simulink model "may7bdrc"  (Simulink 8.5)
settings: Solver=ode4  StartTime=0.0  StopTime=inf  FixedStep=BKIN_STEP_TIME  RelTol=1e-3
StartFcn:
  |  warndlg('Dexterit-E models cannot run under simulation. Please compile your model and run it from within Dexterit-E.');set_param(bdroot,'SimulationCommand','stop')
undefined symbols (not defined in the file): slselsubs
libraries: Video x7, General x3, KINARM_loads x2, KINARM_EP_loads x1, KINARM_general x1, simulink x1, slrtlib x1
(part 2 of 3)

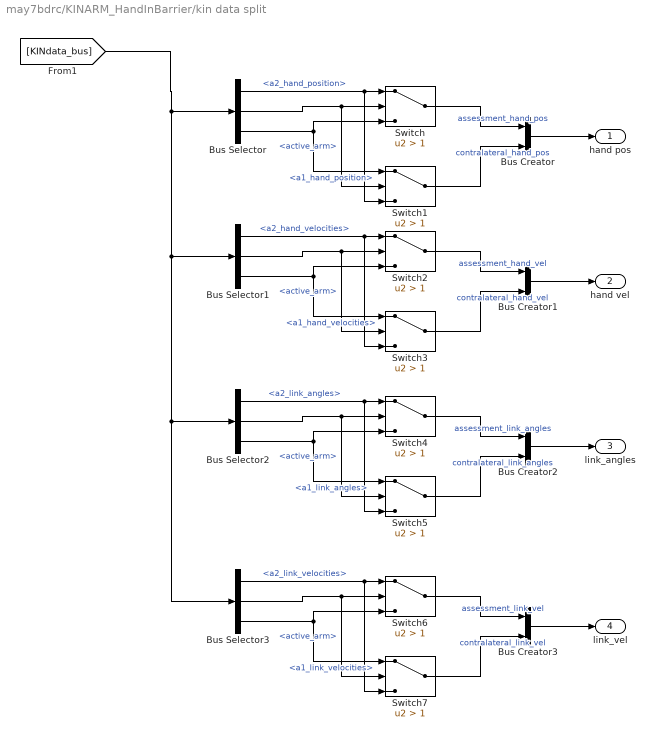
== system may7bdrc/KINARM_HandInBarrier/kin data split ==
  Bus Creator{,1..3} (4 alike) : BusCreator  Inputs=2
  Bus Selector : BusSelector  OutputSignals=Robot2.a2_hand_position,KINDataGeneral.active_arm,Robot1.a1_hand_position
  Bus Selector1 : BusSelector  OutputSignals=Robot2.a2_hand_velocities,KINDataGeneral.active_arm,Robot1.a1_hand_velocities
  Bus Selector2 : BusSelector  OutputSignals=Robot2.a2_link_angles,KINDataGeneral.active_arm,Robot1.a1_link_angles
  Bus Selector3 : BusSelector  OutputSignals=Robot2.a2_link_velocities,KINDataGeneral.active_arm,Robot1.a1_link_velocities
  Switch{,1..7} (8 alike) : Switch  Criteria=u2 > Threshold  Threshold=1
  hand pos : Outport
  hand vel : Outport  Port=2
  link_angles : Outport  Port=3
  link_vel : Outport  Port=4
  wires:
  Bus Selector/1 -> Switch1/3, Switch/1  "<a2_hand_position>"
  Switch/1 -> Bus Creator/1  "assessment_hand_pos"
  Switch1/1 -> Bus Creator/2  "contralateral_hand_pos"
  Bus Creator/1 -> hand pos/1
  Bus Selector/3 -> Switch1/1, Switch/3  "<a1_hand_position>"
  Bus Selector/2 -> Switch1/2, Switch/2  "<active_arm>"
  Bus Selector1/1 -> Switch3/3, Switch2/1  "<a2_hand_velocities>"
  Switch2/1 -> Bus Creator1/1  "assessment_hand_vel"
  Switch3/1 -> Bus Creator1/2  "contralateral_hand_vel"
  Bus Creator1/1 -> hand vel/1
  Bus Selector1/3 -> Switch3/1, Switch2/3  "<a1_hand_velocities>"
  Bus Selector1/2 -> Switch3/2, Switch2/2  "<active_arm>"
  Bus Selector2/1 -> Switch5/3, Switch4/1  "<a2_link_angles>"
  Switch4/1 -> Bus Creator2/1  "assessment_link_angles"
  Switch5/1 -> Bus Creator2/2  "contralateral_link_angles"
  Bus Creator2/1 -> link_angles/1
  Bus Selector2/3 -> Switch5/1, Switch4/3  "<a1_link_angles>"
  Bus Selector2/2 -> Switch5/2, Switch4/2  "<active_arm>"
  Bus Selector3/1 -> Switch7/3, Switch6/1  "<a2_link_velocities>"
  Switch6/1 -> Bus Creator3/1  "assessment_link_vel"
  Switch7/1 -> Bus Creator3/2  "contralateral_link_vel"
  Bus Creator3/1 -> link_vel/1
  [KINdata_bus] -> Bus Selector3/1, Bus Selector2/1, Bus Selector1/1, Bus Selector/1
  Bus Selector3/3 -> Switch7/1, Switch6/3  "<a1_link_velocities>"
  Bus Selector3/2 -> Switch7/2, Switch6/2  "<active_arm>"

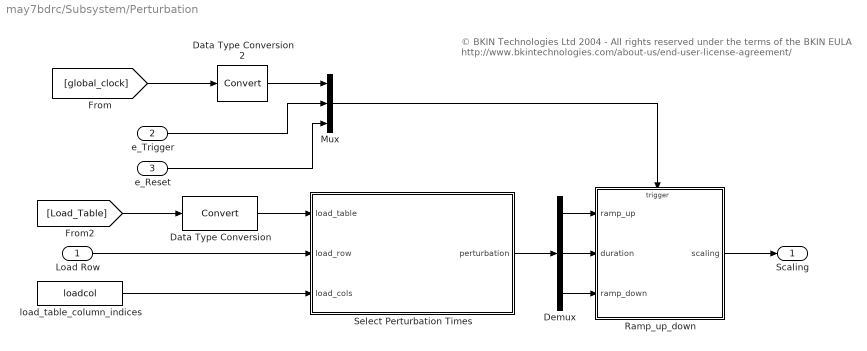
== system may7bdrc/Subsystem/Perturbation ==
  note: © BKIN Technologies Ltd 2004  - All rights reserved under the terms of the BKIN EULA
      | http://www.bkintechnologies.com/about-us/end-user-license-agreement/
  Load Row : Inport
  e_Trigger : Inport  Port=2
  e_Reset : Inport  Port=3
  Data Type Conversion : DataTypeConversion
  Data Type Conversion2 : DataTypeConversion
  Demux : Demux  Outputs=3
  Mux : Mux  Inputs=3
  Ramp_up_down : Stateflow chart  TreatAsAtomicUnit=on
      settings: PermitHierarchicalResolution=ParametersOnly
  Select Perturbation Times : MATLAB Function  TreatAsAtomicUnit=on
      settings: PermitHierarchicalResolution=ParametersOnly
  load_table_column_indices : Constant  Value=loadcol
  Scaling : Outport
  wires:
  Data Type Conversion2/1 -> Mux/1
  Mux/1 -> Ramp_up_down/Trigger
  Demux/3 -> Ramp_up_down/3(ramp_down)
  Demux/2 -> Ramp_up_down/2(duration)
  Demux/1 -> Ramp_up_down/1(ramp_up)
  [global_clock] -> Data Type Conversion2/1
  Ramp_up_down/1(scaling) -> Scaling/1
  e_Trigger/1 -> Mux/2
  e_Reset/1 -> Mux/3
  [Load_Table] -> Data Type Conversion/1
  Load Row/1 -> Select Perturbation Times/2(load_row)
  load_table_column_indices/1 -> Select Perturbation Times/3(load_cols)
  Select Perturbation Times/1(perturbation) -> Demux/1
  Data Type Conversion/1 -> Select Perturbation Times/1(load_table)

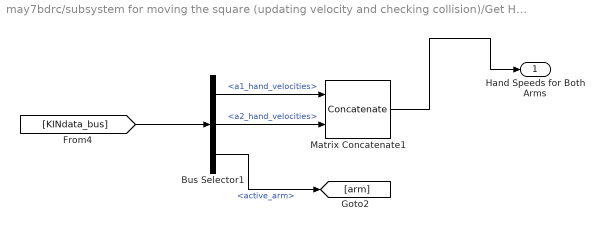
== system may7bdrc/subsystem for moving the square (updating velocity and checking collision)/Get Hand Speed ==
  Bus Selector1 : BusSelector  OutputSignals=Robot1.a1_hand_velocities,Robot2.a2_hand_velocities,KINDataGeneral.active_arm
  Matrix Concatenate1 : Concatenate  Mode=Multidimensional array
  Hand Speeds for Both Arms : Outport
  wires:
  [KINdata_bus] -> Bus Selector1/1
  Bus Selector1/1 -> Matrix Concatenate1/1  "<a1_hand_velocities>"
  Matrix Concatenate1/1 -> Hand Speeds for Both Arms/1
  Bus Selector1/2 -> Matrix Concatenate1/2  "<a2_hand_velocities>"
  Bus Selector1/3 -> [arm]  "<active_arm>"

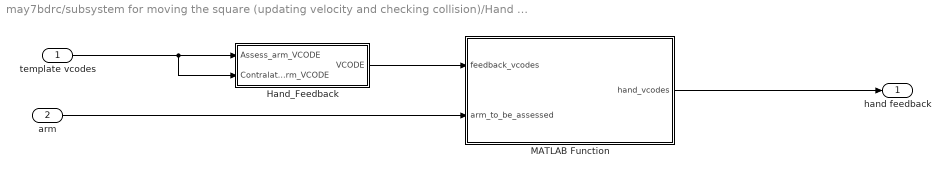
== system may7bdrc/subsystem for moving the square (updating velocity and checking collision)/Hand Feedback ==
  template vcodes : Inport
  arm : Inport  Port=2
  Hand_Feedback : Subsystem  AncestorBlock=KINARM_general/Hand_Feedback  mask(Hand_Feedback){feedback_cntl_src=style and status}
      mask prompts: feedback_cntl_src "Task Program control of style and status"
      mask help:
      | This block controls various options for hand feedback (i.e. fingertip position)  to be shown to the subject.
      |
      | Task Program control of style and status refers to whether the Program Task will explicity control the style and/or status of the hand feedback.
      mask init:
      | block_path = gcb;  % store block path, as gcb may change with block operations
      | 
      | %%% Handle background colours if link status changes.  
      | checkBackgroundColour(block_path, 'KINARM_general');
      | 
      | 
      | feedback_cntl_source=get_param(gcb,'feedback_cntl_src');
      | 
      | if feedback_cntl_source(1:4)=='none'
      |     block1type='Constant';
      |     block2type='Constant';
      |     block3type='Constant';
      | elseif feedback_cntl_source(1:4)=='stat'
      |     block1type='Constant';
      |     block2type='Constant';
      |     block3type='Inport';
      | else 
      |     block1type='Inport';
      |     block2type='Inport';
      |     block3type='Constant';
      | end
      | 
      | hasOldName1 = ~isempty(find_system(gcb, 'FollowLinks', 'on', 'LookUnderMasks', 'all', 'name', 'Dom_VCODE'));
      | hasOldName2 = ~isempty(find_system(gcb, 'FollowLinks', 'on', 'LookUnderMasks', 'all', 'name', 'non-Dom_VCODE'));
      | 
      | block1name='Assess_arm_VCODE';
      | block2name='Contralateral_arm_VCODE';
      | block1path=[gcb '/' block1name];
      | block2path=[gcb '/' block2name];
      | 
      | if hasOldName1
      | 	set_param([gcb '/Dom_VCODE'],'name', block1name);
      | end
      | 
      | if hasOldName2
      | 	set_param([gcb '/non-Dom_VCODE'],'name', block2name);
      | end
      | 
      | if ~strcmp(get_param(block1path,'blocktype'),block1type)
      | 	pos=get_param(block1path,'position');
      | 	delete_line(gcb, [block1name '/1'], 'Reshape/1');
      | 	delete_block(block1path);
      | 	add_block(['built-in/' block1type], block1path,'Name',block1name);
      | 	set_param(block1path,'position',pos);
      | 	add_line(gcb, [block1name '/1'], 'Reshape/1');
      | end
      | 
      | if ~strcmp(get_param(block2path,'blocktype'),block2type)
      | 	pos=get_param(block2path,'position');
      | 	delete_line(gcb, [block2name '/1'], 'Reshape1/1');
      | 	delete_block(block2path);
      | 	add_block(['built-in/' block2type],block2path,'Name',block2name);
      | 	set_param(block2path,'position',pos);
      | 	add_line(gcb, [block2name '/1'], 'Reshape1/1');
      | end
      | 
      | block3name='feedback_status';
      | block3path=[gcb '/' block3name];
      | if ~strcmp(get_param(block3path,'blocktype'),block3type)
      | 	pos=get_param(block3path,'position');
      | 	delete_line(gcb, [block3name '/1'], 'FeedFwdArm/3');
      | 	delete_block(block3path);
      | 	add_block(['built-in/' block3type],block3path,'Name',block3name);
      | 	set_param(block3path,'position',pos);
      | 	add_line(gcb, [block3name '/1'], 'FeedFwdArm/3');
      | end
      | 
      | if feedback_cntl_source(1:4)=='none'
      | 	set_param(block1path,'Value','[1:70]');
      | 	set_param(block2path,'Value','[71:140]');
      | elseif feedback_cntl_source(1:4)=='stat'
      | 	set_param(block1path,'Value','[1:70]');
      | 	set_param(block2path,'Value','[71:140]');
      | end
      mask Help:
      | Creates VCODE for drawing hand position (fingertip).
      | <P>
      | <H2>Library </H2>
      | KINARM general
      | 
      | <H2>Description </H2>
      | This block controls various options for drawing hand feedback.  (Note: although it is called hand feedback, it is actually the fingertip position that is shown).  Three options are available (as chosen in the Parameters and Dialog box):
      | <P>
      | (i) GUI control of feedback style and status
      | <Blockquote>
      | No inputs are required for this option.  The Task Program has no control over the style or status of the hand feedback.
      | </Blockquote>
      | (ii) Task Program control of feedback status and GUI control of style
      | <Blockquote>
      | If Task Program control of feedback status is chosen, then one input appears for this block:<P>
      | <B> feedback_status: </B> this scalar input dynamically controls the status of the hand feedback as per the following:
      | <P>
      | 0 = (no hand feedback)<BR>
      | 1 = ("arm to be assessed" hand feedback only)<BR>
      | 2 = (contralateral arm hand feedback only)<BR>
      | 3 = (hand feedback on for both hands)<BR>
      | </Blockquote>
      | (iii) Task Program control of both feedback style and status.
      | <Blockquote>
      | 
      | If Task Program control of feedback status and style is chosen, then two inputs appear for this block:<P>
      | <B> Assess_arm_VCODE: </B>  this vector input dynamically controls the status and style of the hand feedback for the "arm to be assessed" the operator selected in Dexterit-E.
      | <P>
      | <B> Contralateral_arm_VCODE:</B>  this vector input dynamically controls the status and style of the hand feedback for the contralateral hand.
      | <P>
      | For both the Assess_arm_VCODE and the Contralateral_arm_VCODE, the input vectors must be in the appropriate VCODE format (for more information on the details of a VCODE, please right click on the Show_Target block in the video library, "Look Under Mask" and open the Embedded Matlab function).  Note that the position information in the Dom_VCODE and non-Dom_VCODE are overwritten in this block, but all other aspects of the VCODE are passed through to the output.
      | </Blockquote>
      | Note that if Task Program control is chosen for either hand feedback status or style, the GUI will still override these settings if the Task Protocol specifies that it should do so.
      | <P>
      | There is one output from this block:
      | <P>
      | <B> VCODE: </B> this output is 2-row matrix containing 2 VCODEs.  The first VCODE is for the dominant hand feedback and the second VCODE is for the non-dominant hand feedback.  This output must go to the Process_Video_CMD block of the video library for the hand feedback to actually be shown (if any other visual targets are to be displayed, then this VCODE output must be concatenated with the other VCODES prior to connection to the Process_Video_CMD block - see Help for the Process_Video_CMD block for more information).
      | <H2>Parameters and Dialog Box</H2>
      | <B>Task Program control of style and status</B> refers to whether the Program Task will explicity control the style and/or status of the hand feedback.  The three options are: none, status only, or status and style.
      | <P>
      |  - Choosing none means that style and status are always controlled by the GUI.
      | <P>
      |  - Choosing status only means that the GUI always controls the hand feedback style, but also will create an input to this block allowing the end user to control the status dynamically.  Allowable input values are: 0 (no hand feedback), 1 (dominant hand feedback only), 2 (non-dominant hand feedback only) or 3 (hand feedback on for both hands)
      |  <P>
      | - Choosing status and style means that both the hand feedback status and style can be controlled dynamically by the Task Program.  If this option is selected, then two inputs will be created for this block: dominant VCODE and non-dominant VCODE.  These two inputs require a proper VCODE (e.g. from a Show_Target block) for each.  Because status and style are both part of a VCODE, there is no separate input for hand feedback status.  Note: any position information of these input VCODEs is overwritten by this block by the appropriate fingertip locations.
      | <P>
      | 
      | <H2>Related Blocks </H2>
      | DataLogging<BR>
      | Show_Target<BR>
      | Process_Video_CMD
      mask TypeOptions feedback_cntl_src: none | status only | style and status
  MATLAB Function : MATLAB Function  TreatAsAtomicUnit=on
      settings: PermitHierarchicalResolution=ParametersOnly
  hand feedback : Outport
  wires:
  template vcodes/1 -> Hand_Feedback/2(Contralateral_arm_VCODE), Hand_Feedback/1(Assess_arm_VCODE)
  Hand_Feedback/1(VCODE) -> MATLAB Function/1(feedback_vcodes)
  arm/1 -> MATLAB Function/2(arm_to_be_assessed)
  MATLAB Function/1(hand_vcodes) -> hand feedback/1

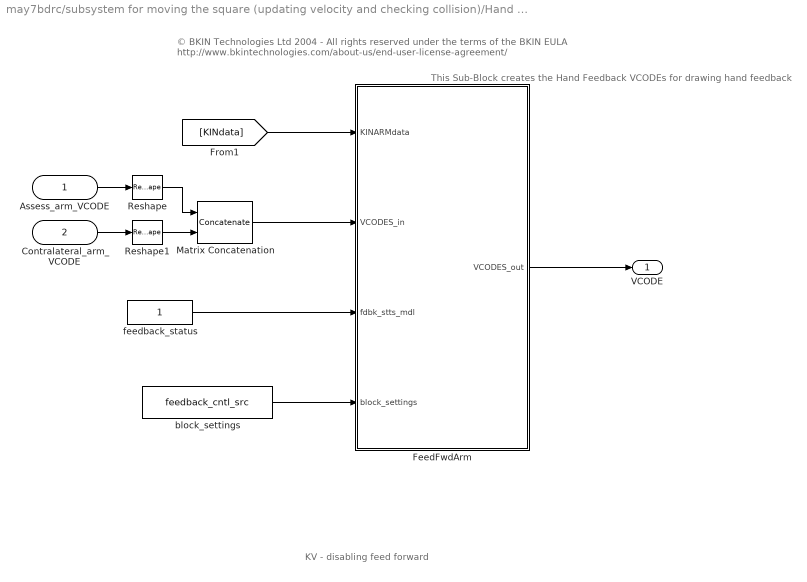
== system may7bdrc/subsystem for moving the square (updating velocity and checking collision)/Hand Feedback/Hand_Feedback ==
  note: KV - disabling feed forward
  note: This Sub-Block creates the Hand Feedback VCODEs for drawing hand feedback
  note: © BKIN Technologies Ltd 2004  - All rights reserved under the terms of the BKIN EULA
      | http://www.bkintechnologies.com/about-us/end-user-license-agreement/
  Assess_arm_VCODE : Inport
  Contralateral_arm_VCODE : Inport  Port=2
  FeedFwdArm : MATLAB Function  TreatAsAtomicUnit=on
      settings: PermitHierarchicalResolution=ParametersOnly  RTWSystemCode=Nonreusable function  RTWFileNameOpts=Use function name
  Matrix Concatenation : Concatenate  Mode=Multidimensional array
  Reshape : Reshape  OutputDimensionality=Row vector (2-D)
  Reshape1 : Reshape  OutputDimensionality=Row vector (2-D)
  block_settings : Constant  Value=feedback_cntl_src
  feedback_status : Constant
  VCODE : Outport
  wires:
  feedback_status/1 -> FeedFwdArm/3(fdbk_stts_mdl)
  FeedFwdArm/1(VCODES_out) -> VCODE/1
  block_settings/1 -> FeedFwdArm/4(block_settings)
  Matrix Concatenation/1 -> FeedFwdArm/2(VCODES_in)
  [KINdata] -> FeedFwdArm/1(KINARMdata)
  Reshape1/1 -> Matrix Concatenation/2
  Reshape/1 -> Matrix Concatenation/1
  Assess_arm_VCODE/1 -> Reshape/1
  Contralateral_arm_VCODE/1 -> Reshape1/1

== stateflow chart subsystem for moving the square (updating velocity and checking collision)/Collision Resolution ==
  settings: sampleTime=0.001
  state Initialize/
    % Stateflow starts here when task is loaded
    entry: force_scaling = [0 0 0 0];
    rect_target_out = zeros(1,70);
    rect_vel = [0 0];
    rect_offset_position = [0 0];
    trial_step = 0;
    trial_stop = 0;
  state Moving_Targets_and_Colliding_Them
    %there are 4 parallel states here. They each execute in the same cycle but in a specific order (see top right of the state)
    % state 3 is the important one - it simply says "move the square according to its velocity"
    % states 1 and 2 check collisions to update that velocity before we get to state 3
    % state 4 then checks to see if we ended up outside the screen and if so, to take us back to the start position
    state CollisionWithHand/ [parallel]
      % this substate will handle collision checks between hands and the square
      settings: executionOrder=1
      state StartWithSpeed0/
        %
        entry:  rect_vel = [0 0];
        rect_offset_position = [0 0];
      state WaitForCollision/
        entry: % state where we wait for collisions to happen
        force_scaling = [0 0 0 0];
        during:
        rect_target_out = rect_target;
        rect_offset_position = rect_offset_position + rect_vel;
        rect_target_out(3:4) = rect_target_out(3:4)+rect_offset_position
        target_colliding = check_collision(circ_target, rect_target, rect_offset_position)
      state ResolveTargetCollision
        during: % if something collided, we're going to separate the two objects and then use elastic collision to update velocities
        % eject the rectangle
        rect_offset_position = eject( circ_target( target_colliding,:), rect_target, rect_offset_position);
        prev_vel = rect_vel;
        hand_vel = hand_speed( target_colliding,:)/1e3;
        % elastic collision equations - here m = 1 and is the same for hand and square. It is used here to provide relative mass
        % between the two objects. The forces here will be further multiplied by a fudge factor (see the Simulink forces section)
        rect_vel(1) = (mr - mc)/(mr + mc)*rect_vel(1) + 2*mc/(mc + mr)*hand_vel(1);
        rect_vel(2) = (mr - mc)/(mr + mc)*rect_vel(2) + 2*mc/(mc + mr)*hand_vel(2);
        hand_vector = [1 2; 3 4];
        % a bump will be generated that will be proportional to change in velocity
        force_scaling(hand_vector(target_colliding,:)) = prev_vel - rect_vel;
      WaitForCollision -> StartWithSpeed0 [order 2] : e_Trial_Start
      StartWithSpeed0 -> WaitForCollision
      WaitForCollision -> ResolveTargetCollision [order 1] : [ target_colliding]
      ResolveTargetCollision -> WaitForCollision : [~check_collision(circ_target( target_colliding,:), rect_target, rect_offset_position)]
          | /{target_colliding=0}
    state CollisionWithWall/ [parallel] [commented out]
      % this substate will handle collision between square and screen edges.
      % is the rectangle at the left edge of the screen
      en, du: if((rect_target_out(3)-rect_target_out(10)/2) < -display_size(1)/2)
      %rect_vel(1) = -rect_vel(1);
      trial_step = 2
      rect_vel(1) = 0;
      end
      % is the rectangle at the right edge of the screen
      if((rect_target_out(3)+rect_target_out(10)/2) > display_size(1)/2)
      %rect_vel(1) = -rect_vel(1);
      trial_step = 2
      rect_vel(1) = 0;
      end
      % is the rectangle at top of the scren
      if((rect_target_out(4)+rect_target_out(11)/2) > display_size(2))
      %rect_vel(2) = -rect_vel(2);
      trial_step = 2
      rect_vel(2) = 0;
      end
      % is the rectangle at bottom of the scren
      if((rect_target_out(4)-rect_target_out(11)/2) < 0)
      trial_step = 2
      rect_vel(2) = 0;
      %rect_vel(2) = -rect_vel(2);
      end
    state PositionUpdated/ [parallel]
      % once collision is handled, move the square by its velocity
      during: rect_target_out = rect_target;
      rect_offset_position = rect_offset_position + rect_vel;
      rect_target_out(3:4) = rect_target_out(3:4)+rect_offset_position;
      settings: executionOrder=2
    state CheckToSeeIfGoalReached1/ [parallel] [commented out]
      % once the participant hits the square (denoted by the puck), then we want to calculate if it is inside of the goal or not. this is done using the input form prior matrix.
      % since the input ot this block is the vcode, we access the dimesnion of the vector that contains length., width, height. in the start position with 0 velocity
      % Get rectangle (puck) info
      rect_x = rect_target_out(3);
      rect_y = rect_target_out(4);
      rect_w = rect_target_out(10);
      rect_h = rect_target_out(11);
      % Get goal info
      goal_x = goal_target(3);
      goal_y = goal_target(4);
      goal_w = goal_target(10);
      goal_h = goal_target(11);
      % Compute edges
      rect_left   = rect_x - rect_w / 2;
      rect_right  = rect_x + rect_w / 2;
      rect_top    = rect_y + rect_h / 2;
      rect_bottom = rect_y - rect_h / 2;
      goal_left   = goal_x - goal_w / 2;
      goal_right  = goal_x + goal_w / 2;
      goal_top    = goal_y + goal_h / 2;
      goal_bottom = goal_y - goal_h / 2;
      % Check for full puck in goal (fully inside goal)
      if (rect_left >= goal_left) && (rect_right <= goal_right) && ...
      (rect_bottom >= goal_bottom) && (rect_top <= goal_top)
      % Fully inside goal
      trial_step = 3;
      trial_stop = 1;
      %rect_vel = [0, 0];  % Stop motion
      %rect_offset_position = [0, 0];  % Optionalreset
      end
    state CheckToSeeIfWeAreOutofBounds1/ [parallel] [commented out]
      % once everything is done moving and colliding, we check to see if we're off the screen still. If we are, put the square in the start position with 0 velocity
      % once collision is handled, move the square by its velocity
      % Reset everything as soon as the rectangle touches the side of the screen
      during:
      if (rect_target_out(3) - rect_target_out(10)/2 <= -display_size(1)/2) || ...
      (rect_target_out(3) + rect_target_out(10)/2 >= display_size(1)/2) || ...
      (rect_target_out(4) + rect_target_out(11)/2 >= display_size(2)) || ...
      (rect_target_out(4) - rect_target_out(11)/2 <= 0)
      % Reset all movement variables
      rect_vel = [0, 0];  % Stop movement
      rect_offset_position = [0, 0];  % Reset position
      trial_step = 4;
      trial_stop = 1;  % Set flag to stop trial
      end
  (default) -> Initialize
  Initialize -> StartWithSpeed0
  data: colliding_target function_output double; circ_matrix_in function_input double; rect_vector_in function_input double; rect_offset_in function_input double; eject_rect_offset function_output double; circ_vcode_in function_input double; rect_vcode_in function_input double; rect_offset function_input double; trial_protocol input double; circ_target input double; circ_to_barrier_target input double; rect_target_out output double size=[1 70]; rect_target input double; barrier_target input double size=[1 70]; display_size input double; force_scaling output double; mc input double; mr input double; hand_vector local double; rect_vel local double; prev_vel local double; target_colliding local double; hand_vel local double; rect_offset_position local double; trial_stop output double size=[1]; goal_target input double; trial_step output double; mb input double size=1; barrier_colliding local double; hand_speed input double; check_collision_barrier1 local double; barrier_vel local double; force_scaling_barrier local double; rect_y local double; rect_w local double; rect_h local double; rect_x local double; goal_h local double; goal_y local double; goal_w local double; goal_x local double; rect_top local double; goal_top local double; hand_offset_position local double; prev_hand_vel local double; rect_left local double; rect_bottom local double; goal_right local double; rect_right local double; goal_bottom local double; goal_left local double; new_hand_posistion_c local double
  events: e_clk input RISING_EDGE_EVENT; e_Trial_Start input EITHER_EDGE_EVENT; e_Trial_Start1 input EITHER_EDGE_EVENT
  function colliding_target = check_collision(circ_matrix_in, rect_vector_in, rect_offset_in):
    | function colliding_target = check_collision(circ_matrix_in, rect_vector_in, rect_offset_in)
    | 
    | % calculates collision between 2 circles (ie. either hand feedback) and rectangle
    | % inputs:
    | %        circ_matrix_in - 2x70 matrix that is 2 circle vcodes
    | %        rect_vector_in - 1x70 vector that is a rectangle vcode
    | %        rect_offset_in - position offset for rect_vector_ in to calculate
    | %                         where the rectangle is
    | % outputs:
    | %        colliding_target values:
    | %              0- if nothing colliding
    | %              1- if rectangle collided with right hand
    | %              2- if rectangle colliding with left hand
    | 
    | x = 3;
    | y = 4;
    | 
    | colliding_target = 0;
    | 
    | for ii = 1:size(circ_matrix_in,1)
    | 	
    | 	current_circle_vcode = circ_matrix_in(ii,:);
    | 	
    | 	radius = current_circle_vcode(10);
    | 	w = rect_vector_in(10);
    | 	h = rect_vector_in(10);
    | 	
    | 	x0 = current_circle_vcode(x);
    | 	y0 = current_circle_vcode(y);
    | 	
    | 	X0 = rect_vector_in(x)+rect_offset_in(1);
    | 	Y0 = rect_vector_in(y)+rect_offset_in(2);
    | 	
    | 	deltax = x0-X0;
    | 	deltay = y0-Y0;
    | 	
    | 	w = rect_vector_in(10);  %width (sizes in cm in v1.4)
    | 	h = rect_vector_in(11);  %height (sizes in cm in v1.4)
    | 	
    | 	t = rect_vector_in(12)/180*pi;
    | 	
    | 	sint=sin(t);
    | 	cost=cos(t);
    | 	
    | 	xrotate=deltax.*cost + deltay.*sint;   %location of x point in rectangle's coordinate frame
    | 	yrotate=-deltax.*sint + deltay.*cost;  %location of y point in rectangle's coordinate frame
    | 		
    | 	%intarget = (abs(xrotate) < (w/2+radius)) & (abs(yrotate) < (h/2+radius));
    | 	
    | 	%--------------%
    | 	DeltaX = xrotate - max(0 - w/2, min(xrotate, 0 + w/2));
    | 	DeltaY = yrotate - max(0 - h/2, min(yrotate, 0 + h/2));
    | 	intarget = 1*(DeltaX * DeltaX + DeltaY * DeltaY) < (radius * radius);
    | 	
    | 	%--------------%
    | 	
    | 	
    | 	if intarget
    | 		colliding_target = ii;
    | 		break;
    | 	end
    | 	
    | end
  function eject_rect_offset = eject(circ_vcode_in, rect_vcode_in, rect_offset):
    | function eject_rect_offset = eject(circ_vcode_in, rect_vcode_in, rect_offset)
    | 
    | % moves the rectangle_vcode out of a circle_vcode if the two are
    | % overlapping
    | 
    | x = 3;
    | y = 4;
    | 
    | radius = circ_vcode_in(10);
    | w = rect_vcode_in(10);
    | h = rect_vcode_in(10);
    | 
    | x0 = circ_vcode_in(x);
    | y0 = circ_vcode_in(y);
    | 
    | X0 = rect_vcode_in(x)+rect_offset(1);
    | Y0 = rect_vcode_in(y)+rect_offset(2);
    | 
    | deltax = x0-X0;
    | deltay = y0-Y0;
    | 
    | w = rect_vcode_in(10);  %width (sizes in cm in v1.4)
    | h = rect_vcode_in(11);  %height (sizes in cm in v1.4)
    | 
    | t = rect_vcode_in(12)/180*pi;
    | 
    | sint=sin(t);
    | cost=cos(t);
    | 
    | xrotate=deltax.*cost + deltay.*sint;   %location of x point in rectangle's coordinate frame
    | yrotate=-deltax.*sint + deltay.*cost;  %location of y point in rectangle's coordinate frame
    | 
    | % so xrotate and yrotate is where the circle is inside the rectangle
    | theta_threshold = atan(h / w); % get the threshold - angles below this go out the side while angles
    | % above this go out the top
    | 
    | % calculating magnitude
    | 
    | % polar coordinate to the circle
    | [t_c, ~] = cart2pol(abs(xrotate), abs(yrotate));
    | 
    | if t_c < theta_threshold % the rectangle will be moved along its local x-axis to exit the circle
    |     x_eject_local = (w/2+radius-abs(xrotate))*sign(-xrotate); % if the circle is on the right, move the rectangle left and vice-versa
    |     y_eject_local = 0;
    | else % going out top/bottom % the rectangle will be moved along its local y-axis to exit the circle
    |     x_eject_local = 0;
    |     y_eject_local = (h/2+radius-abs(yrotate))*sign(-yrotate); % if the circle is above the rectangle, move the rectangle down and vice-versa
    | end
    | 
    | % convert the local offsets to global coordinates by undoing the rotation
    | 
    | % rotate back to global coordinates
    | sint=sin(-t);
    | cost=cos(-t);
    | 
    | x_eject_global = x_eject_local.*cost + y_eject_local.*sint;   
    | y_eject_global = - x_eject_local.*sint + y_eject_local.*cost;
    | 
    | eject_rect_offset = rect_offset + [x_eject_global y_eject_global];

== matlab function subsystem for moving the square (updating velocity and checking collision)/Hand Feedback/MATLAB Function ==
  data: feedback_vcodes input double; arm_to_be_assessed input double; hand_vcodes output double
function hand_vcodes = fcn(feedback_vcodes, arm_to_be_assessed)
% the hand feedback vcodes are sorted like this:
%    <arm to be assessed vcode>
%    <contralateral arm> 
% but using this function I am going to sort the vcodes like this:
%    <right arm>
%    <left arm>
% because that will make it easier to track velocities and forces

if arm_to_be_assessed == 1
	hand_vcodes = feedback_vcodes;
else
	hand_vcodes = feedback_vcodes([2 1], :);
	%hand_vcodes = feedback_vcodes;
end

== stateflow chart Trial_Control ==
  settings: sampleTime=0.001
  state Initialize/
    % Set variables
    entry:
    logging_enable = true;
    start_target_row = Trial_Protocol(START_ROW);
    preshot_area_row = Trial_Protocol(PRESHOT_ROW);
    cursor_row = Trial_Protocol(CIRCLE_ROW);
    puck_row = Trial_Protocol(RECT_ROW);
    barrier_target_row = Trial_Protocol(BARRIER_ROW);
    goal_target_row = Trial_Protocol(GOAL_ROW);
    load_row = Trial_Protocol(LOAD_ROW);
    trial_duration = Trial_Protocol(SECONDS);
    start_hold_time = Trial_Protocol(START_HOLD_TIME);
    shot_ready_time = Trial_Protocol(SHOT_READY_TIME);
    shot_set_time = Trial_Protocol(SHOT_SET_TIME);
    goal_time = Trial_Protocol(GOAL_TIME);
  state Main_Trial/
    % Each trial task only initializes variables and then runs for Trial_Protocol(SECONDS) seconds before stopping
    state StartHold/
      entry:
      start_target_state = 3;
      preshot_area_state=0;
      puck_state=0;
      goal_target_state=0;
      barrier_target_state=0;
      event_code = E_ENTER_START_AREA;
    state PreshotStart/
      % send e_Trial_End event
      entry:
      preshot_area_state=3;
      puck_state=2;
      goal_target_state=2;
      barrier_target_state=2;
      event_code = E_ENTER_PRESHOT_AREA;
    state StartOn/
      entry:
      start_target_state = 2;
      preshot_area_state = 0;
      cursor_state = 2;
      puck_state = 0;
      barrier_target_state = 0;
      goal_target_state = 0;
      e_Trial_Start;
      event_code = E_TRIAL_BEGIN;
    state PreshotMove/
      % send e_Trial_End event
      entry:
    state ShotReady/
      % send e_Trial_End event
      entry:
      event_code = E_EXIT;
    state ShotSet/
      % send e_Trial_End event
      entry:
      preshot_area_state=0;
    state Success/
      % send e_Trial_End event
      entry:
      puck_state=0;
      goal_target_state=3
    state PuckInGoal/
      % send e_Trial_End event
      entry:
    state Shot/
      % send e_Trial_End event
      entry:
      start_target_state=0;
    state Fail/
      % send e_Trial_End event
      entry:
      start_target_state=0;
      preshot_area_state = 0;
      cursor_state = 2;
      puck_state = 0;
      barrier_target_state = 0;
      goal_target_state = 0;
    StartHold -> PreshotStart [order 2] : after(start_hold_time,sec)
    StartOn -> StartHold [order 1] : [HandInTarget(start_target_row,1)==1]
    PreshotStart -> PreshotMove [order 2] : [HandInTarget(start_target_row,1)==0]
    StartHold -> StartOn [order 1] : [HandInTarget(start_target_row,1)==0]
    PreshotStart -> StartHold [order 1] : [HandInTarget(preshot_area_row,1)==0]
    ShotSet -> StartOn [order 1] : [HandInTarget(start_target_row,1)==0]
    PreshotMove -> StartOn [order 2] : [HandInTarget(preshot_area_row,1)==0]
    ShotReady -> PreshotMove [order 1] : [HandInTarget(start_target_row,1)==0]
    PreshotMove -> ShotReady [order 1] : [HandInTarget(start_target_row,1)==1]
    ShotReady -> ShotSet [order 2] : after(shot_ready_time,sec)
    ShotSet -> Shot [order 2] : after(shot_set_time,sec)
    PuckInGoal -> Success [order 1] : after(goal_time,sec)
    Shot -> PuckInGoal [order 3] : [PuckInTarget(goal_target_row,1)==1]
    PuckInGoal -> Fail [order 2] : [PuckInTarget(goal_target_row,1)==0]
    Shot -> Fail [order 2] : [HandInBarrier(barrier_target_row,1)==1]
    Shot -> Fail [order 1] : after(trial_duration,sec)
  state Inter_Trial_State/
    % send e_Trial_End event
    entry:
    e_Trial_End;
    event_code = E_TRIAL_ENDED;
  (default) -> Initialize
  Initialize -> StartOn
  Inter_Trial_State -> StartOn : after(1, sec)
  StartOn -> Inter_Trial_State [order 2] : after(trial_duration, sec)
  Main_Trial -> Inter_Trial_State : e_ExitTrialNow
  Fail -> Inter_Trial_State : after(0.3,sec)
  Success -> Inter_Trial_State : after(0.3,sec)
  data: logging_enable output boolean; event_code output double; cursor_row output double; cursor_state output double; puck_row output double; puck_state output double; load_row output double; Trial_Protocol input double; trial_duration local double; barrier_target_row output double; barrier_target_state output double; start_target_row output double; start_target_state output double; goal_target_row output double; goal_target_state output double; HandInTarget input double; trial_ended input double; trial_step_datas input double; preshot_area_state output double; preshot_area_row output double; start_hold_time local double; shot_set_time local double; shot_ready_time local double; HandInBarrier input double; PuckInTarget input double; goal_time local double
  events: e_clk input RISING_EDGE_EVENT; e_ExitTrialNow input EITHER_EDGE_EVENT; e_Trial_End output EITHER_EDGE_EVENT; e_Trial_Start output EITHER_EDGE_EVENT

== matlab function subsystem for moving the square (updating velocity and checking collision)/Hand Feedback/Hand_Feedback/FeedFwdArm ==
  settings: fimath=|
      | fimath(...
      | 'RoundMode', 'floor',...
      | 'OverflowMode', 'wrap',...
      | 'ProductMode', 'KeepLSB', 'ProductWordLength', 32,...
      | 'SumMode', 'KeepLSB', 'SumWordLength', 32,...
      | 'CastBeforeSum', false)
  data: KINARMdata input double; VCODES_in input double; VCODES_out output double; fdbk_stts_mdl input double; block_settings input double
function VCODES_out  = fcn(KINARMdata,VCODES_in,fdbk_stts_mdl, block_settings)
%
% This function creates the VCODEs for the hand position feedback for both
% hands.  Various options in the Mask of the Simulink block in which this
% embedded Matlab file sits, allow the user to specify how often
% the hand feedback is updated as well as the source of the style and status
% of the hand feedback.  
%
% block_settings is the value chosen by the user in the Mask for parent Simulink
% block.  Note: that even if the block is wired up to accept Task Program 
% control of hand feedback style and status, this embedded Matlab file allows
% the GUI to over-ride those settings.  However, if the GUI requests that
% the parent block use Task Program control for the style and/or status when
% it has not been programmed in, then this embedded Matlab file handles this
% appropriately and ignore the request for Task Program control.  
%
% block_settings=1 -- parent block does not have any Task Program control over style or status
% block_settings=2 -- parent block has Task Program control over status only
% block_settings=3 -- parent block has Task Program control over both style and status
%
% fdbk_stts_mdl (only potentially used if block_settings=2) 
% fdbk_stts_mdl=0 -- neither hand on
% fdbk_stts_mdl=1 -- dominant hand on
% fdbk_stts_mdl=2 -- non-dominant hand on
% fdbk_stts_mdl=3 -- both hands on
%
% VCODES (only potentially used if block_settings=3) 
% VCODES for dominant and non-dominant, input to parent block 


dominant_arm=KINARMdata(3,1);
feedfwd=KINARMdata(3,2);				%amount of feedforward extrapolation for hand position(s)
fdbk_stts_GUI=KINARMdata(3,3);			%status of hand feedback requested from GUI
fdbk_src_GUI=KINARMdata(3,4);			%source of hand feedback style requested from GUI
fdbk_clr_GUI=KINARMdata(3,5);			%colour of hand feedback required by GUI
fdbk_radius_GUI=KINARMdata(3,6);		%radius of hand feedback required by GUI


%----------------Feedback Style ----------------
% IF GUI asks for feedback style from Task Program (fdbk_src_GUI==0)
% AND if Task Program has been chosen to supply feedback style (block_settings==3)
% AND if Task Program actually supplies appropriate feedback styles (size(VCODES_in,2)==70)
if fdbk_src_GUI==0 && block_settings==3 && size(VCODES_in,2)==70
    VCODES=VCODES_in;
else
    VCODES=zeros(2,70);						%set default
	VCODES(:,1)=1;							%target_type of circle
	VCODES(:,5)=fdbk_clr_GUI;				%fill colour as specified by GUI
	VCODES(:,6)=fdbk_clr_GUI;				%stroke colour same as fill colour
	VCODES(:,7)=0;							%no stroke width
    VCODES(:,9)=100.0;                      %100% opacity
	VCODES(:,10)=fdbk_radius_GUI;			%radius (m) as specified by GUI
end

%----------------Feedback Status ----------------
%feedback status from GUI sets the default to be used
feedback_status=fdbk_stts_GUI;


if fdbk_stts_GUI==4				%if GUI has requested Task Program control of feedback status
	if block_settings==2		%if there is Task Program control ONLY of status (but not style)
		feedback_status=fdbk_stts_mdl;		%then use feedback status input from parent block
	elseif block_settings==3	%if there is Task Program control of both status and style
		feedback_status=4;		%then let the input VCODEs handle the status
	else						%otherwise assume that the Task Program did not provide style OR status
		feedback_status=3;		%then set both hands are always on as a default
    end
else		%if GUI is controlling feedback status
	feedback_status=fdbk_stts_GUI;
end

%set the status of the hand-feedback in the VCODES
switch feedback_status
	case 0					%show neither hand feedback
		VCODES(1,2)=0;
		VCODES(2,2)=0;
	case 1					%show ONLY dominant hand feedback
		VCODES(1,2)=1;
		VCODES(2,2)=0;
	case 2					%show ONLY non-dominant hand feedback
		VCODES(1,2)=0;
		VCODES(2,2)=1;
	case 4					%VCODES already control hand feedback
		%do nothing
	otherwise				%show both hand feedbacks
		VCODES(1,2)=1;
		VCODES(2,2)=1;
end

%----------------Feedback Position ----------------
%set the position of the hand feedback.
for i=1:2
	if i==1
		active_arm=KINARMdata(3,1);			%choose dominant arm first
	else
		active_arm=3-KINARMdata(3,1);		%choose non-dominant arm 2nd
	end
	HandXPos=KINARMdata(active_arm,23);		%(m)
	HandYPos=KINARMdata(active_arm,24);		%(m)
	HandXVel=KINARMdata(active_arm,25);		%(m/s)
	HandYVel=KINARMdata(active_arm,26);		%(m/s)

	% feed-forward hand position (m)
	%HandXPos_ff = HandXPos + HandXVel*feedfwd;
	%HandYPos_ff = HandYPos + HandYVel*feedfwd;
	HandXPos_ff = HandXPos;
	HandYPos_ff = HandYPos;
	VCODES(i,3)=HandXPos_ff;				%target position in m 
	VCODES(i,4)=HandYPos_ff;				%target position in m 
end

VCODES_out=VCODES;

== matlab function PuckInTarget/Embedded MATLAB InsideTarget ==
  settings: fimath=|
      | fimath(...
      | 'RoundMode', 'floor',...
      | 'OverflowMode', 'wrap',...
      | 'ProductMode', 'KeepLSB', 'ProductWordLength', 32,...
      | 'SumMode', 'KeepLSB', 'SumWordLength', 32,...
      | 'CastBeforeSum', false)
  data: handpos input double size=2; target_type input double; attribcol input double; num_targets input double; intarget output double; Target_Table input double
function intarget = FIsInsideTarget(handpos, target_type, attribcol, num_targets, Target_Table)
% all dimensions in m, rad
% arguments:
% handpos: x,y positions of center of target
% attribcol: columns in target table specifying target attributes.  
% Specific to Target_Type
%	circle:
%	[X0,Y0,r...,rn] where:
%	X0,Y0 : centre of circle
%	r : logical radius of circle (i.e. radius used to determine 'in' or 'out' of target)
%	rn: logical radius of other targets (e.g. 2nd, 3rd) also specified in target row.
%   Up to 4 targets can be specified in a row
% ellipse:
%	[X0,Y0,a,b,t...,an, bn, tn] where:
%	X0,Y0 : centre of ellipse
%	a,b : major, minor radii of ellipse
%	t : rotation of ellipse in degrees
%	an,bn : major, minor radii of ellipse of other targets (e.g. 2nd, 3rd) also specified in target row
%	tn : rotation of ellipse in degrees of other targets (e.g. 2nd, 3rd) also specified in target row
%   Up to 4 targets can be specified in a row


target_col_x=1;
target_col_y=2;

x=handpos(1);
y=handpos(2);

intarget = zeros(size(Target_Table,1),5);

X0 = Target_Table(:,target_col_x)*0.01;			%Target Table sizes in cm in v1.4
Y0 = Target_Table(:,target_col_y)*0.01;			%Target Table sizes in cm in v1.4

deltax=x-X0;
deltay=y-Y0;

if target_type==1			%circle
	for target=1:num_targets
		r = Target_Table(:,attribcol(target))*0.01;			%Target Table sizes in cm in v1.4
		% simple euclidean distance
		distance2 = deltax.^2 + deltay.^2;					%distance2 is the square of the distance
	    intarget(:,target) = (distance2 <= r.^2);
	end
elseif target_type==2		%ellipse
	for target=1:num_targets
	    a = Target_Table(:,attribcol(target*3-2))*0.01;			%Target Table sizes in cm in v1.4
	    b = Target_Table(:,attribcol(target*3-1))*0.01;			%Target Table sizes in cm in v1.4	
	    t = Target_Table(:,attribcol(target*3))*(pi / 180.0);	%Target Table angles in degrees in v1.4
		sint=sin(t);
		cost=cos(t);
		xrotate=deltax.*cost+deltay.*sint;		%location of x point in ellipse's coordinate frame
		yrotate=-deltax.*sint+deltay.*cost;		%location of y point in ellipse's coordinate frame
		m=yrotate./xrotate;						%slope of line between the (x,y) to (x0,y0) in ellipse's coordinate frame
		y2sq=1./(1./(m.*a).^2+1./b.^2);			%y2sq is y2^2, where y2 is the intersection of the ellipse and the (x,y) to (x0,y0) line
	    intarget(:,target) = (yrotate.^2 <= y2sq);
    end
elseif target_type==3       %rectangle
    for target=1:num_targets
        w = Target_Table(:,attribcol(target*3-2))*0.01;  %width (sizes in cm in v1.4)
        h = Target_Table(:,attribcol(target*3-1))*0.01;  %height (sizes in cm in v1.4)
        
        if attribcol(target*3) > 0
            t = Target_Table(:,attribcol(target*3))*(pi / 180.0);  %angle (angles in degrees in v1.4)
        else
            t = zeros(size(Target_Table, 1), 1);
        end

        sint=sin(t);
        cost=cos(t);

        xrotate=deltax.*cost + deltay.*sint;   %location of x point in rectangle's coordinate frame
        yrotate=-deltax.*sint + deltay.*cost;  %location of y point in rectangle's coordinate frame

        intarget(:,target) = abs(xrotate) <= w/2 & abs(yrotate) <= h/2;
    end
elseif target_type==4       %line
    for target=1:num_targets
        % treat the line like a rectangle of height h and width w
        % determine height (stroke width) in the same fashion as in Show_Target
        if attribcol(target*3-2) == 0                     %0 column index means stroke width of 0
            h = zeros(size(Target_Table, 1), 1);
        elseif attribcol(target*3-2) < 0                  %-ve column index means stroke width of 1mm
            h = ones(size(Target_Table, 1), 1) .* 0.001;
        else
            h = Target_Table(:,attribcol(target*3-2)) * 0.01;  %target table contains width in cm
        end
        
        ex = Target_Table(:,attribcol(target*3-1))*0.01;  %endpoint in x relative to start point (cm)
        ey = Target_Table(:,attribcol(target*3))*0.01;    %endpoint in y relative to start point (cm)
        
        w = sqrt(ex.^2 + ey.^2);                          %width (cm)
        
        % determine the vector from the line's midpoint to the hand position
        handx = deltax - ex/2;
        handy = deltay - ey/2;
        
        t = atan2(ey, ex);                                %calculate angle of the line (rads)
        sint = sin(t);
        cost = cos(t);
        
        xrotate = handx.*cost + handy.*sint;   %location of x point in rectangle's coordinate frame
        yrotate = -handx.*sint + handy.*cost;  %location of y point in rectangle's coordinate frame
 
        intarget(:,target) = abs(xrotate) <= w/2 & abs(yrotate) <= h/2;
    end
elseif target_type==5  % triangle
    for target=1:num_targets
        w = Target_Table(:,attribcol(target*4-3))*0.01;         %length (sizes in cm in v1.4)
        
        % If a height column of 0 is specified, make the triangle equilateral. Otherwise, use the
        % values for height and peak offset from the target table.
        if attribcol(target*4-2) > 0
            h = Target_Table(:,attribcol(target*4-2))*0.01;  %height (sizes in cm in v1.4)
            p = Target_Table(:,attribcol(target*4-1))*0.01;  %peak offset (sizes in cm in v1.4)
        else
            h = w.*sin(pi/3.0);
            p = zeros(size(Target_Table, 1), 1);
        end
        
        if attribcol(target*4) > 0
            t = Target_Table(:,attribcol(target*4))*(pi / 180.0);  %angle (angles in degrees in v1.4)
        else
            t = zeros(size(Target_Table, 1), 1);
        end
        
        sint = sin(t);
        cost = cos(t);
        
        xrotate = deltax.*cost + deltay.*sint;   %location of x point in triangle's coordinate frame
        yrotate = -deltax.*sint + deltay.*cost;  %location of y point in triangle's coordinate frame
        
        % Perform a point-in-triangle test using Barycentric coordinates.
        A = [-w/2 - p/3, -h/3];
        B = [2*p/3, 2*h/3];
        C = [w/2 - p/3, -h/3];
        
        v0 = C - A;
        v1 = B - A;
        v2 = [xrotate, yrotate] - A;

        dot00 = v0(:,1) .* v0(:,1) + v0(:,2) .* v0(:,2);
        dot01 = v0(:,1) .* v1(:,1) + v0(:,2) .* v1(:,2);
        dot02 = v0(:,1) .* v2(:,1) + v0(:,2) .* v2(:,2);
        dot11 = v1(:,1) .* v1(:,1) + v1(:,2) .* v1(:,2);
        dot12 = v1(:,1) .* v2(:,1) + v1(:,2) .* v2(:,2);

        invDenom = 1 ./ (dot00 .* dot11 - dot01 .* dot01);
        u = (dot11 .* dot02 - dot01 .* dot12) .* invDenom;
        v = (dot00 .* dot12 - dot01 .* dot02) .* invDenom;

        intarget(:,target) = (u > 0) & (v > 0) & (u + v < 1);
    end
end
